simulink model "airship"  (Simulink 7.5)
settings: Solver=ode45  StartTime=0.0  StopTime=2  RelTol=1e-3
values from neighbouring files (symbols this model uses):
  a1 = 5    [valuables.m]
  a2 = 2*a1    (= 10)    [valuables.m]
  b = 3.7/2    (= 1.85)    [valuables.m]
  bottom = 0    [valuables.m]
  CL1 = (1/2)*DiffCLZeta*Sf*Nf*Lf3    (= 2.0002634928)    [valuables.m]
  CL2 = -Cdcg*Sg*Lgz    (= -1.344)    [valuables.m]
  CM1 = K21*Nk*Sh*I2*L    (= 217.968531349)    [valuables.m]
  CM2 = (-1/2)*DiffCLAlpha*Sf*Nf*Lf1    (= -59.34811401)    [valuables.m]
  CM3 = -((Cdch*J2*Sh*L)+(Cdcf*Sf*Lf2))    (= -168.6714915)    [valuables.m]
  CM4 = (-1/2)*DiffCLZeta*Sf*Nf*Lf1    (= -12.84322188)    [valuables.m]
  CX1 = -(Cdh0*Sh+Cdf0*Sf+Cdg0*Sg)    (= -0.6313245)    [valuables.m]
  CY1 = K21*Nk*Sh*I1    (= -6.9497212894)    [valuables.m]
  CY2 = (-1/2)*DiffCLAlpha*Sf*Nf    (= -8.4181722)    [valuables.m]
  CY3 = -((Cdch*J1*Sh)+(Cdcf*Sf)+(Cdcg*Sg))    (= -25.4932315)    [valuables.m]
  CY4 = (-1/2)*DiffCLZeta*Sf*Nf    (= -1.8217336)    [valuables.m]
  CZ3 = -((Cdch*J1*Sh)+(Cdcf*Sf))    (= -24.9332315)    [valuables.m]
  del = (Ixx*Izz)-(Ixz*Ixz)    (= 676199)    [valuables.m]
  g = 0.0669    [valuables.m]
  h0 = 200    [valuables.m]
  Ixx = 213    [valuables.m]
  Ixz = 88    [valuables.m]
  Iyy = 3310    [valuables.m]
  Izz = 3211    [valuables.m]
  left = 0    [valuables.m]
  mass = 136.8    [valuables.m]
  right = 0    [valuables.m]
  TL = 0.3    [valuables.m]
  top = 0    [valuables.m]
  TR = 0.3    [valuables.m]
  TS = 0.3    [valuables.m]
  u0 = 10    [valuables.m]
  XL = 8.13    [valuables.m]
  Xs = 12.5    [valuables.m]
  YL = 0.6    [valuables.m]
  ZL = 0.2    [valuables.m]
  Zs = 0.25    [valuables.m]
libraries: vrlib x2
settings Model: Creator=knightofaccess  LastModifiedBy=ex08148

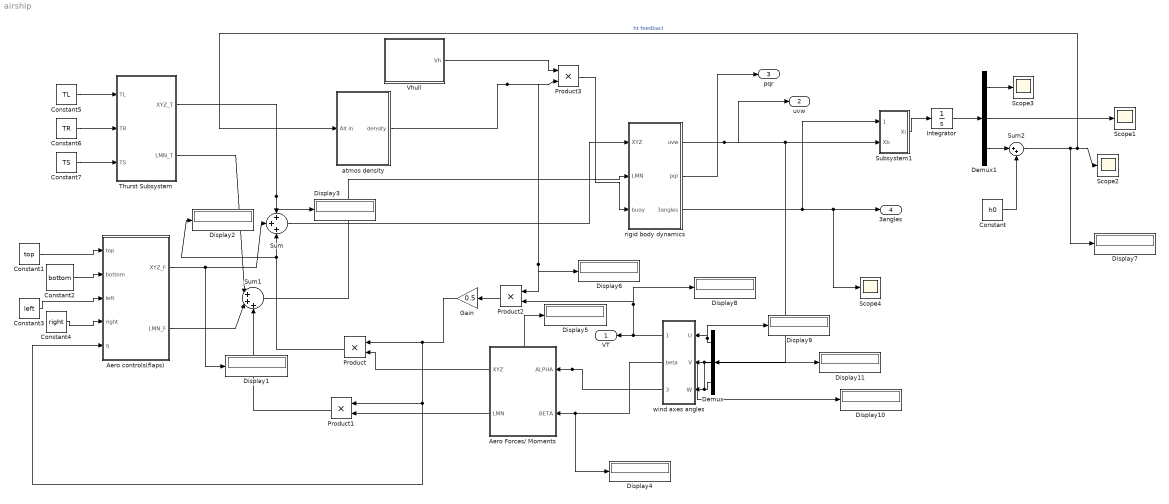
== system airship ==
  Aero Forces/ Moments : Subsystem
  Aero controls(flaps) : Subsystem
  Constant : Constant  Value=h0  OutDataType=fixdt(1, 16)  OutScaling=2^0
  Constant1 : Constant  Value=top  OutDataType=fixdt(1, 16)  OutScaling=2^0
  Constant2 : Constant  Value=bottom  OutDataType=fixdt(1, 16)  OutScaling=2^0
  Constant3 : Constant  Value=left  OutDataType=fixdt(1, 16)  OutScaling=2^0
  Constant4 : Constant  Value=right  OutDataType=fixdt(1, 16)  OutScaling=2^0
  Constant5 : Constant  Value=TL  OutDataType=fixdt(1, 16)  OutScaling=2^0
  Constant6 : Constant  Value=TR  OutDataType=fixdt(1, 16)  OutScaling=2^0
  Constant7 : Constant  Value=TS  OutDataType=fixdt(1, 16)  OutScaling=2^0
  Demux : Demux  Outputs=3
  Demux1 : Demux  Outputs=3
  Display{1..11} (11 alike) : Display
  Gain : Gain  Gain=0.5  ParameterDataType=fixdt(1, 16)  ParameterScaling=2^0  OutDataType=fixdt(1, 16)  OutScaling=2^0
  Integrator : Integrator
  Product{,1..3} (4 alike) : Product  OutDataType=fixdt(1, 16)  OutScaling=2^0  RndMeth=Zero
  Scope{1..4} (4 alike) : Scope
      Scope2 settings: SaveName=ScopeData2
      Scope4 settings: SaveName=ScopeData3
  Subsystem1 : Subsystem
  Sum : Sum  Inputs=+++  OutDataType=fixdt(1, 16)  OutScaling=2^0
  Sum1 : Sum  Inputs=|+++  OutDataType=fixdt(1, 16)  OutScaling=2^0
  Sum2 : Sum  Inputs=|++  OutDataType=fixdt(1, 16)  OutScaling=2^0
  Thurst Subsystem : Subsystem
  Vhull : Subsystem
  atmos density : Subsystem
  rigid body dynamics : Subsystem
  wind axes angles : Subsystem
  VT : Outport  OutDataType=fixdt(1, 16)  OutScaling=2^0
  uvw : Outport  Port=2
  pqr : Outport  Port=3
  3angles : Outport  Port=4
  wires:
  Thurst Subsystem/1(XYZ_T) -> Sum/1, Display3/1
  Thurst Subsystem/2(LMN_T) -> Sum1/1
  Constant5/1 -> Thurst Subsystem/1(TL)
  Constant6/1 -> Thurst Subsystem/2(TR)
  Constant7/1 -> Thurst Subsystem/3(TS)
  Aero controls(flaps)/2(LMN_F) -> Sum1/2
  Constant1/1 -> Aero controls(flaps)/1(top)
  Constant2/1 -> Aero controls(flaps)/2(bottom)
  Constant3/1 -> Aero controls(flaps)/3(left)
  Constant4/1 -> Aero controls(flaps)/4(right)
  Aero controls(flaps)/1(XYZ_F) -> Sum/2, Display1/1
  Aero Forces/ Moments/1(XYZ) -> Product/2
  Aero Forces/ Moments/2(LMN) -> Product1/2
  Product1/1 -> Sum1/3
  Product/1 -> Sum/3, Display2/1
  Demux/1 -> wind axes angles/1(U), Display9/1
  Demux/2 -> wind axes angles/2(V), Display10/1
  wind axes angles/1(VT*VT) -> VT/1, Product2/2, Display8/1
  wind axes angles/2(beta) -> Aero Forces/ Moments/2(BETA), Display4/1
  wind axes angles/3(alpha) -> Aero Forces/ Moments/1(ALPHA), Display5/1
  Product2/1 -> Gain/1
  Gain/1 -> Product/1, Aero controls(flaps)/5(q), Product1/1
  rigid body dynamics/1(uvw) -> uvw/1, Subsystem1/2(Xb), Demux/1
  rigid body dynamics/2(pqr) -> pqr/1
  Sum/1 -> rigid body dynamics/1(XYZ)
  Sum1/1 -> rigid body dynamics/2(LMN)
  rigid body dynamics/3(3angles) -> Subsystem1/1(3angles), 3angles/1, Scope4/1
  Vhull/1(Vh) -> Product3/1
  atmos density/1(density) -> Product3/2, Product2/1, Display6/1
  Product3/1 -> rigid body dynamics/3(buoy)
  Demux/3 -> wind axes angles/3(W), Display11/1
  Subsystem1/1(Xi) -> Integrator/1
  Integrator/1 -> Demux1/1
  Demux1/1 -> Scope3/1
  Demux1/2 -> Scope1/1
  Demux1/3 -> Sum2/1
  Constant/1 -> Sum2/2
  Sum2/1 -> atmos density/1(Alt in), Scope2/1, Display7/1  "ht feedbacl"

== system airship/Aero Forces/ Moments ==
  ALPHA : Inport  OutDataType=sfix(16)  OutScaling=2^0
  BETA : Inport  Port=2  OutDataType=sfix(16)  OutScaling=2^0
  Subsystem : Subsystem
  Subsystem1 : Subsystem
  XYZ : Outport  OutDataType=sfix(16)  OutScaling=2^0
  LMN : Outport  Port=2  OutDataType=sfix(16)  OutScaling=2^0
  wires:
  Subsystem/1(XYZ) -> XYZ/1
  Subsystem1/1(LMN) -> LMN/1
  ALPHA/1 -> Subsystem/1(ALPHA), Subsystem1/2(ALPHA)  "ALPHA"
  BETA/1 -> Subsystem/2(BETA), Subsystem1/1(BETA)  "BETA"

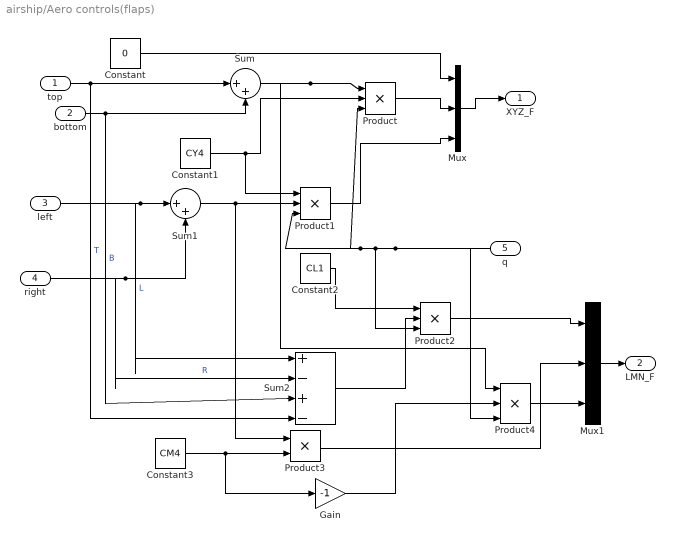
== system airship/Aero controls(flaps) ==
  top : Inport  OutDataType=sfix(16)  OutScaling=2^0
  bottom : Inport  Port=2  OutDataType=sfix(16)  OutScaling=2^0
  left : Inport  Port=3  OutDataType=sfix(16)  OutScaling=2^0
  right : Inport  Port=4  OutDataType=sfix(16)  OutScaling=2^0
  q : Inport  Port=5  OutDataType=fixdt(1, 16)  OutScaling=2^0
  Constant : Constant  Value=0  OutDataType=sfix(16)  OutScaling=2^0
  Constant1 : Constant  Value=CY4  OutDataType=sfix(16)  OutScaling=2^0
  Constant2 : Constant  Value=CL1  OutDataType=sfix(16)  OutScaling=2^0
  Constant3 : Constant  Value=CM4  OutDataType=sfix(16)  OutScaling=2^0
  Gain : Gain  Gain=-1  ParameterDataType=sfix(16)  ParameterScaling=2^0  OutDataType=sfix(16)  OutScaling=2^0
  Mux : Mux  Inputs=3
  Mux1 : Mux  Inputs=3
  Product{,1..2,4} (4 alike) : Product  Inputs=3  OutDataType=sfix(16)  OutScaling=2^0  RndMeth=Zero
  Product3 : Product  OutDataType=sfix(16)  OutScaling=2^0  RndMeth=Zero
  Sum : Sum  Inputs=|++  OutDataType=sfix(16)  OutScaling=2^0
  Sum1 : Sum  Inputs=|++  OutDataType=sfix(16)  OutScaling=2^0
  Sum2 : Sum  Inputs=|+-+-  OutDataType=sfix(16)  OutScaling=2^0
  XYZ_F : Outport  OutDataType=sfix(16)  OutScaling=2^0
  LMN_F : Outport  Port=2  OutDataType=sfix(16)  OutScaling=2^0
  wires:
  top/1 -> Sum/1, Sum2/4  "T"
  bottom/1 -> Sum/2, Sum2/3  "B"
  Sum/1 -> Product/1, Product4/1
  Constant1/1 -> Product/2, Product1/1
  left/1 -> Sum1/1, Sum2/1  "L"
  right/1 -> Sum1/2, Sum2/2  "R"
  Sum1/1 -> Product1/2, Product3/1
  Constant/1 -> Mux/1
  Product/1 -> Mux/2
  Product1/1 -> Mux/3
  Sum2/1 -> Product2/2
  Constant2/1 -> Product2/1
  Constant3/1 -> Product3/2, Gain/1
  Product4/1 -> Mux1/3
  Product3/1 -> Mux1/2
  Product2/1 -> Mux1/1
  Mux1/1 -> LMN_F/1
  Gain/1 -> Product4/2
  q/1 -> Product1/3, Product/3, Product4/3, Product2/3
  Mux/1 -> XYZ_F/1

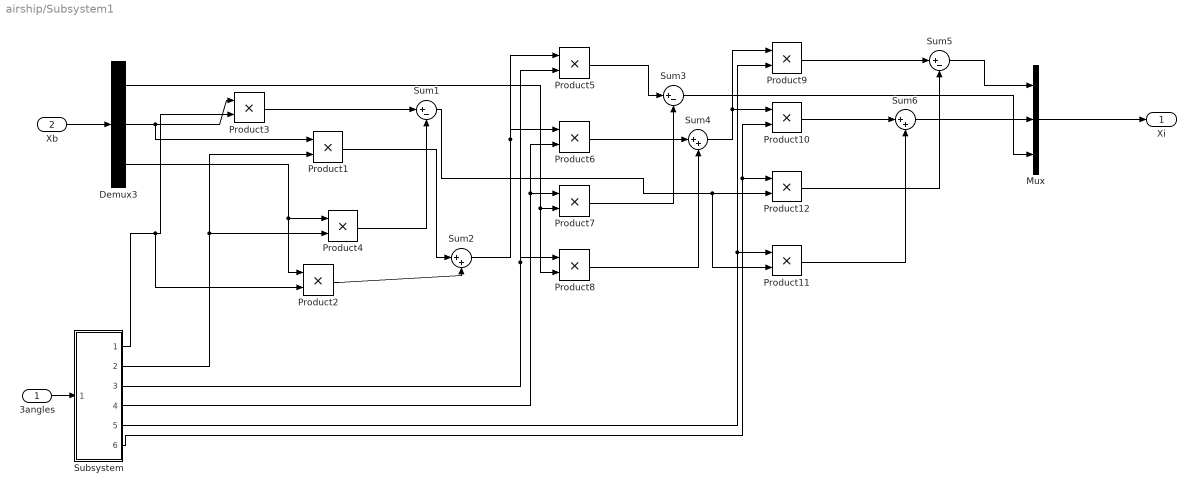
== system airship/Subsystem1 ==
  3angles : Inport  OutDataType=sfix(16)  OutScaling=2^0
  Xb : Inport  Port=2  OutDataType=sfix(16)  OutScaling=2^0
  Demux3 : Demux  Outputs=3
  Mux : Mux  Inputs=3
  Product{1..12} (12 alike) : Product  OutDataType=fixdt(1, 16)  OutScaling=2^0  RndMeth=Zero
  Subsystem : Subsystem
  Sum1 : Sum  Inputs=|+-  OutDataType=fixdt(1, 16)  OutScaling=2^0
  Sum2 : Sum  Inputs=|++  OutDataType=fixdt(1, 16)  OutScaling=2^0
  Sum3 : Sum  Inputs=|+-  OutDataType=fixdt(1, 16)  OutScaling=2^0
  Sum4 : Sum  Inputs=|++  OutDataType=fixdt(1, 16)  OutScaling=2^0
  Sum5 : Sum  Inputs=|+-  OutDataType=fixdt(1, 16)  OutScaling=2^0
  Sum6 : Sum  Inputs=|++  OutDataType=fixdt(1, 16)  OutScaling=2^0
  Xi : Outport  OutDataType=fixdt(1, 16)  OutScaling=2^0
  wires:
  3angles/1 -> Subsystem/1(3angles)
  Xb/1 -> Demux3/1
  Demux3/2 -> Product3/1, Product1/1
  Subsystem/1(cphi) -> Product3/2, Product2/2
  Subsystem/2(sphi) -> Product1/2, Product4/2
  Demux3/3 -> Product2/1, Product4/1
  Product4/1 -> Sum1/2
  Product2/1 -> Sum2/2
  Product3/1 -> Sum1/1
  Product1/1 -> Sum2/1
  Sum2/1 -> Product5/1, Product6/1
  Subsystem/3(ctheta) -> Product5/2, Product8/1
  Subsystem/4(stheta) -> Product6/2, Product7/1
  Demux3/1 -> Product7/2, Product8/2
  Product5/1 -> Sum3/1
  Product7/1 -> Sum3/2
  Product6/1 -> Sum4/1
  Product8/1 -> Sum4/2
  Sum4/1 -> Product9/1, Product10/1
  Subsystem/5(cpsi) -> Product9/2, Product11/1
  Subsystem/6(spsi) -> Product10/2, Product12/1
  Sum1/1 -> Product12/2, Product11/2
  Product9/1 -> Sum5/1
  Product12/1 -> Sum5/2
  Product10/1 -> Sum6/1
  Product11/1 -> Sum6/2
  Sum5/1 -> Mux/1
  Sum6/1 -> Mux/2
  Sum3/1 -> Mux/3
  Mux/1 -> Xi/1

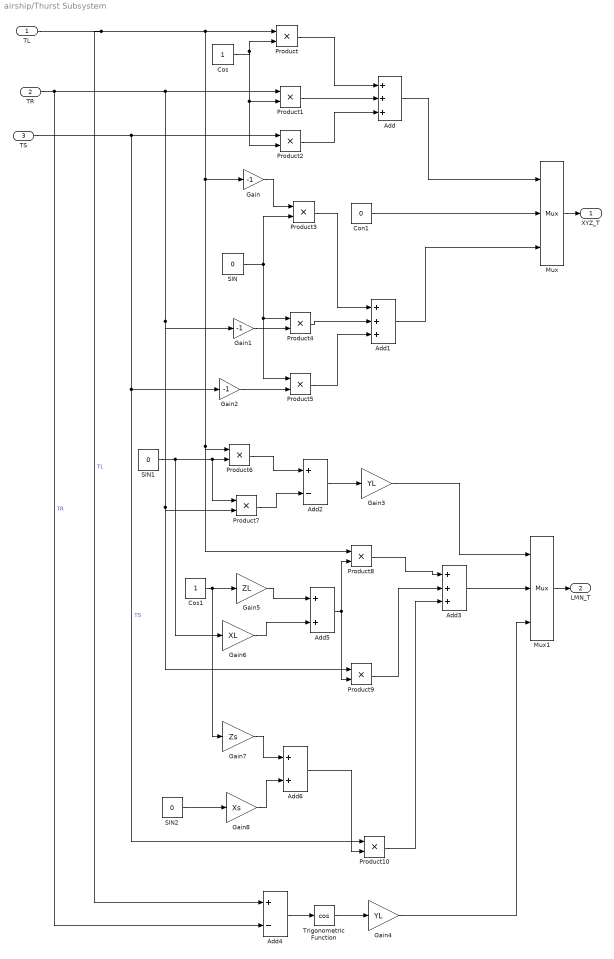
== system airship/Thurst Subsystem ==
  TL : Inport  OutDataType=sfix(16)  OutScaling=2^0
  TR : Inport  Port=2  OutDataType=sfix(16)  OutScaling=2^0
  TS : Inport  Port=3  OutDataType=sfix(16)  OutScaling=2^0
  Add : Sum  Inputs=+++  OutDataType=sfix(16)  OutScaling=2^-10
  Add1 : Sum  Inputs=+++  OutDataType=sfix(16)  OutScaling=2^-10
  Add2 : Sum  Inputs=+-  OutDataType=sfix(16)  OutScaling=2^-10
  Add3 : Sum  Inputs=+++  OutDataType=sfix(16)  OutScaling=2^-10
  Add4 : Sum  Inputs=+-  OutDataType=sfix(16)  OutScaling=2^-10
  Add5 : Sum  OutDataType=sfix(16)  OutScaling=2^-10
  Add6 : Sum  OutDataType=sfix(16)  OutScaling=2^-10
  Con1 : Constant  Value=0  OutDataType=sfix(16)  OutScaling=2^0
  Cos : Constant  OutDataType=sfix(16)  OutScaling=2^0
  Cos1 : Constant  OutDataType=sfix(16)  OutScaling=2^0
  Gain : Gain  Gain=-1  ParameterDataType=sfix(16)  ParameterScaling=2^0  OutDataType=sfix(16)  OutScaling=2^0
  Gain1 : Gain  Gain=-1  ParameterDataType=sfix(16)  ParameterScaling=2^0  OutDataType=sfix(16)  OutScaling=2^0
  Gain2 : Gain  Gain=-1  ParameterDataType=sfix(16)  ParameterScaling=2^0  OutDataType=sfix(16)  OutScaling=2^0
  Gain3 : Gain  Gain=YL  ParameterDataType=sfix(16)  ParameterScaling=2^0  OutDataType=sfix(16)  OutScaling=2^0
  Gain4 : Gain  Gain=YL  ParameterDataType=sfix(16)  ParameterScaling=2^0  OutDataType=sfix(16)  OutScaling=2^0
  Gain5 : Gain  Gain=ZL  ParameterDataType=sfix(16)  ParameterScaling=2^0  OutDataType=sfix(16)  OutScaling=2^0
  Gain6 : Gain  Gain=XL  ParameterDataType=sfix(16)  ParameterScaling=2^0  OutDataType=sfix(16)  OutScaling=2^0
  Gain7 : Gain  Gain=Zs  ParameterDataType=sfix(16)  ParameterScaling=2^0  OutDataType=sfix(16)  OutScaling=2^0
  Gain8 : Gain  Gain=Xs  ParameterDataType=sfix(16)  ParameterScaling=2^0  OutDataType=sfix(16)  OutScaling=2^0
  Mux : Mux  Inputs=3
  Mux1 : Mux  Inputs=3
  Product{,1..10} (11 alike) : Product  OutDataType=sfix(16)  OutScaling=2^0  RndMeth=Zero
  SIN : Constant  Value=0  OutDataType=sfix(16)  OutScaling=2^0
  SIN1 : Constant  Value=0  OutDataType=sfix(16)  OutScaling=2^0
  SIN2 : Constant  Value=0  OutDataType=sfix(16)  OutScaling=2^0
  Trigonometric Function : Trigonometry  Operator=cos  SampleTime=0
  XYZ_T : Outport  OutDataType=sfix(16)  OutScaling=2^0
  LMN_T : Outport  Port=2  OutDataType=sfix(16)  OutScaling=2^0
  wires:
  TL/1 -> Product/1, Gain/1, Product6/1, Product8/1, Add4/1  "TL"
  Cos/1 -> Product/2, Product1/2, Product2/2
  TR/1 -> Product1/1, Gain1/1, Product7/2, Product9/1, Add4/2  "TR"
  TS/1 -> Product2/1, Gain2/1, Product10/1  "TS"
  Product/1 -> Add/1
  Product1/1 -> Add/2
  Product2/1 -> Add/3
  SIN/1 -> Product3/2, Product4/1, Product5/1
  Gain/1 -> Product3/1
  Gain1/1 -> Product4/2
  Gain2/1 -> Product5/2
  Product3/1 -> Add1/1
  Product4/1 -> Add1/2
  Product5/1 -> Add1/3
  Add/1 -> Mux/1
  Con1/1 -> Mux/2
  Add1/1 -> Mux/3
  SIN1/1 -> Product6/2, Product7/1, Gain6/1
  Product6/1 -> Add2/1
  Product7/1 -> Add2/2
  Add2/1 -> Gain3/1
  Gain3/1 -> Mux1/1
  Product8/1 -> Add3/1
  Product9/1 -> Add3/2
  Product10/1 -> Add3/3
  Add3/1 -> Mux1/2
  Gain4/1 -> Mux1/3
  Mux/1 -> XYZ_T/1
  Mux1/1 -> LMN_T/1
  Gain5/1 -> Add5/1
  Cos1/1 -> Gain5/1, Gain7/1
  Gain6/1 -> Add5/2
  Add5/1 -> Product8/2, Product9/2
  SIN2/1 -> Gain8/1
  Gain7/1 -> Add6/1
  Gain8/1 -> Add6/2
  Add6/1 -> Product10/2
  Trigonometric Function/1 -> Gain4/1
  Add4/1 -> Trigonometric Function/1

== system airship/Vhull ==
  Constant : Constant  Value=a1  OutDataType=sfix(16)  OutScaling=2^0
  Constant1 : Constant  Value=a2  OutDataType=sfix(16)  OutScaling=2^0
  Constant2 : Constant  Value=b*b  OutDataType=sfix(16)  OutScaling=2^0
  Gain : Gain  Gain=pi*2/3  ParameterDataType=sfix(16)  ParameterScaling=2^0  OutDataType=sfix(16)  OutScaling=2^0
  Product : Product  OutDataType=sfix(16)  OutScaling=2^0  RndMeth=Zero
  Subtract : Sum  OutDataType=sfix(16)  OutScaling=2^-10
  Vh : Outport  OutDataType=sfix(16)  OutScaling=2^0
  wires:
  Constant/1 -> Subtract/1
  Constant1/1 -> Subtract/2
  Subtract/1 -> Product/1
  Constant2/1 -> Product/2
  Product/1 -> Gain/1
  Gain/1 -> Vh/1

== system airship/atmos density ==
  Alt in : Inport  OutDataType=sfix(16)  OutScaling=2^0
  Constant : Constant  Value=0.0065  OutDataType=sfix(16)  OutScaling=2^0
  Constant1 : Constant  Value=288.15  OutDataType=sfix(16)  OutScaling=2^0
  Display1 : Display
  Divide1 : Product  Inputs=*/  OutDataType=fixdt(1, 16)  OutScaling=2^-10
  Fcn : Fcn  Expr=u^4.256
  Gain : Gain  Gain=1.22505  ParameterDataType=sfix(16)  ParameterScaling=2^0  OutDataType=sfix(16)  OutScaling=2^0
  Product : Product  OutDataType=sfix(16)  OutScaling=2^0  RndMeth=Zero
  Sum2 : Sum  Inputs=|-+
  density : Outport  OutDataType=sfix(16)  OutScaling=2^0
  wires:
  Constant/1 -> Product/2
  Product/1 -> Sum2/1
  Constant1/1 -> Sum2/2, Divide1/2
  Divide1/1 -> Fcn/1
  Fcn/1 -> Gain/1, Display1/1
  Alt in/1 -> Product/1
  Gain/1 -> density/1
  Sum2/1 -> Divide1/1

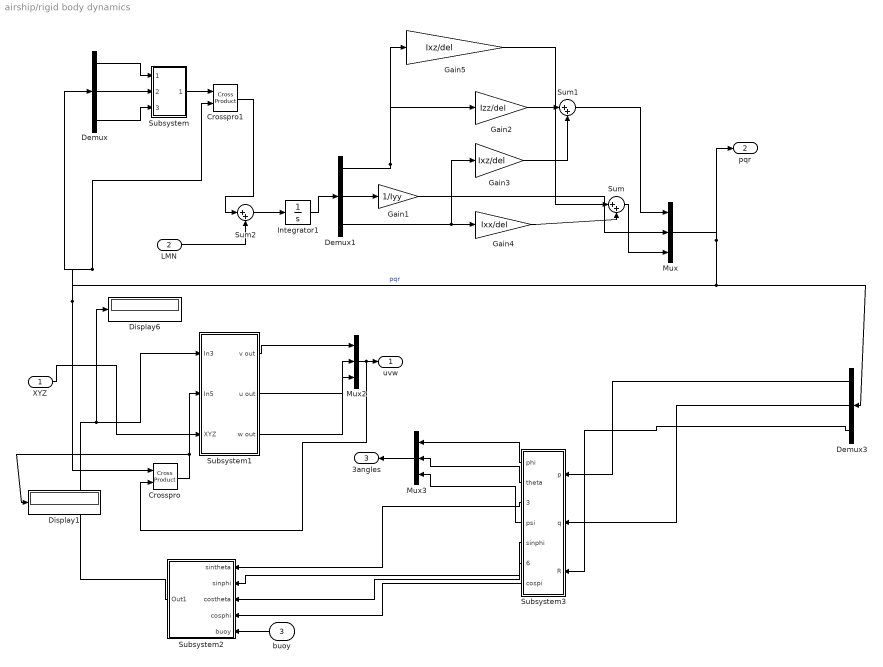
== system airship/rigid body dynamics ==
  XYZ : Inport
  LMN : Inport  Port=2
  buoy : Inport  Port=3
  Crosspro : vrlib/Utilities/Cross Product  SystemSampleTime=-1
  Crosspro1 : vrlib/Utilities/Cross Product  SystemSampleTime=-1
  Demux : Demux  Outputs=3
  Demux1 : Demux  Outputs=3
  Demux3 : Demux  Outputs=3
  Display1 : Display
  Display6 : Display
  Gain1 : Gain  Gain=1/Iyy
  Gain2 : Gain  Gain=Izz/del
  Gain3 : Gain  Gain=Ixz/del
  Gain4 : Gain  Gain=Ixx/del
  Gain5 : Gain  Gain=Ixz/del
  Integrator1 : Integrator
  Mux : Mux  Inputs=3
  Mux2 : Mux  Inputs=3
  Mux3 : Mux  Inputs=3
  Subsystem : Subsystem
  Subsystem1 : Subsystem
  Subsystem2 : Subsystem
  Subsystem3 : Subsystem
  Sum : Sum  Inputs=|++
  Sum1 : Sum  Inputs=|++
  Sum2 : Sum  Inputs=|++
  uvw : Outport
  pqr : Outport  Port=2
  3angles : Outport  Port=3
  wires:
  Mux3/1 -> 3angles/1
  Mux2/1 -> uvw/1, Crosspro/2
  Demux/2 -> Subsystem/2(In2)
  Demux/1 -> Subsystem/1(In1)
  Demux/3 -> Subsystem/3(In3)
  Demux1/1 -> Gain5/1, Gain2/1
  Demux1/2 -> Gain1/1
  Demux1/3 -> Gain4/1, Gain3/1
  Gain4/1 -> Sum/2
  Gain5/1 -> Sum/1
  Gain2/1 -> Sum1/1
  Gain3/1 -> Sum1/2
  Gain1/1 -> Mux/2
  Sum1/1 -> Mux/1
  Sum/1 -> Mux/3
  Mux/1 -> Demux/1, Crosspro1/2, Crosspro/1, Demux3/1, pqr/1  "pqr"
  Subsystem/1(Out1) -> Crosspro1/1
  Crosspro1/1 -> Sum2/1
  Sum2/1 -> Integrator1/1
  Integrator1/1 -> Demux1/1
  Crosspro/1 -> Subsystem1/2(In5), Display1/1
  Subsystem1/1(v out) -> Mux2/1
  Subsystem1/2(u out) -> Mux2/2
  Subsystem1/3(w out) -> Mux2/3
  Subsystem2/1(Out1) -> Subsystem1/1(In3), Display6/1
  Subsystem3/1(phi) -> Mux3/1
  Subsystem3/2(theta) -> Mux3/2
  Demux3/1 -> Subsystem3/1(p)
  Demux3/2 -> Subsystem3/2(q)
  Demux3/3 -> Subsystem3/3(R)
  Subsystem3/3(sinthta) -> Subsystem2/1(sintheta)
  Subsystem3/4(psi) -> Mux3/3
  Subsystem3/6(costhta) -> Subsystem2/3(costheta)
  Subsystem3/7(cospi) -> Subsystem2/4(cosphi)
  Subsystem3/5(sinphi) -> Subsystem2/2(sinphi)
  XYZ/1 -> Subsystem1/3(XYZ)
  LMN/1 -> Sum2/2
  buoy/1 -> Subsystem2/5(buoy)

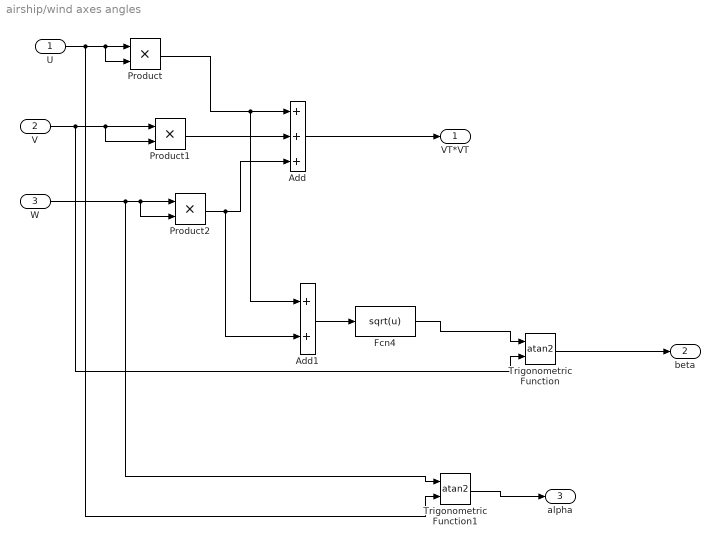
== system airship/wind axes angles ==
  U : Inport  OutDataType=fixdt(1, 16)  OutScaling=2^0
  V : Inport  Port=2  OutDataType=fixdt(1, 16)  OutScaling=2^0
  W : Inport  Port=3  OutDataType=fixdt(1, 16)  OutScaling=2^0
  Add : Sum  Inputs=+++  OutDataType=fixdt(1, 16)  OutScaling=2^-10
  Add1 : Sum  OutDataType=fixdt(1, 16)  OutScaling=2^-10
  Fcn4 : Fcn  Expr=sqrt(u)
  Product : Product  OutDataType=fixdt(1, 16)  OutScaling=2^0  RndMeth=Zero
  Product1 : Product  OutDataType=fixdt(1, 16)  OutScaling=2^0  RndMeth=Zero
  Product2 : Product  OutDataType=fixdt(1, 16)  OutScaling=2^0  RndMeth=Zero
  Trigonometric Function : Trigonometry  Operator=atan2
  Trigonometric Function1 : Trigonometry  Operator=atan2
  VT*VT : Outport  OutDataType=fixdt(1, 16)  OutScaling=2^0
  beta : Outport  Port=2  OutDataType=fixdt(1, 16)  OutScaling=2^0
  alpha : Outport  Port=3  OutDataType=fixdt(1, 16)  OutScaling=2^0
  wires:
  U/1 -> Product/1, Product/2, Trigonometric Function1/2
  V/1 -> Product1/1, Product1/2, Trigonometric Function/2
  W/1 -> Product2/1, Product2/2, Trigonometric Function1/1
  Product/1 -> Add/1, Add1/1
  Product1/1 -> Add/2
  Product2/1 -> Add/3, Add1/2
  Add1/1 -> Fcn4/1
  Fcn4/1 -> Trigonometric Function/1
  Add/1 -> VT*VT/1
  Trigonometric Function1/1 -> alpha/1
  Trigonometric Function/1 -> beta/1

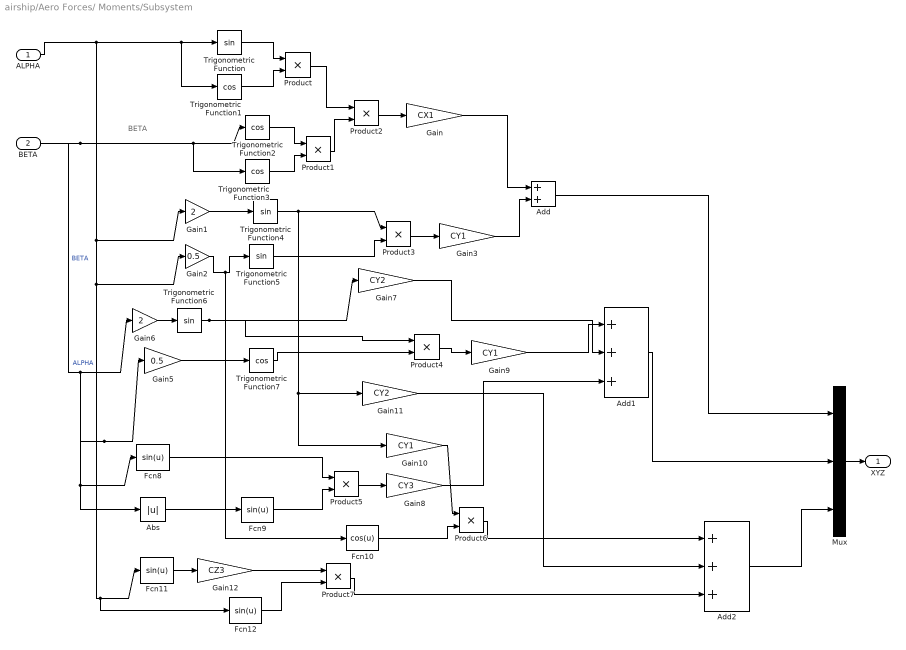
== system airship/Aero Forces/ Moments/Subsystem ==
  note: BETA
  ALPHA : Inport  OutDataType=sfix(16)  OutScaling=2^0
  BETA : Inport  Port=2  OutDataType=sfix(16)  OutScaling=2^0
  Abs : Abs
  Add : Sum  OutDataType=sfix(16)  OutScaling=2^-10
  Add1 : Sum  Inputs=+++  OutDataType=sfix(16)  OutScaling=2^-10
  Add2 : Sum  Inputs=+++  OutDataType=sfix(16)  OutScaling=2^-10
  Fcn10 : Fcn  Expr=cos(u)
  Fcn{8..9,11..12} (4 alike) : Fcn  Expr=sin(u)
  Gain : Gain  Gain=CX1  ParameterDataType=sfix(16)  ParameterScaling=2^0  OutDataType=sfix(16)  OutScaling=2^0
  Gain1 : Gain  Gain=2  ParameterDataType=sfix(16)  ParameterScaling=2^0  OutDataType=sfix(16)  OutScaling=2^0
  Gain10 : Gain  Gain=CY1  ParameterDataType=sfix(16)  ParameterScaling=2^0  OutDataType=sfix(16)  OutScaling=2^0
  Gain11 : Gain  Gain=CY2  ParameterDataType=sfix(16)  ParameterScaling=2^0  OutDataType=sfix(16)  OutScaling=2^0
  Gain12 : Gain  Gain=CZ3  ParameterDataType=sfix(16)  ParameterScaling=2^0  OutDataType=sfix(16)  OutScaling=2^0
  Gain2 : Gain  Gain=0.5  ParameterDataType=sfix(16)  ParameterScaling=2^0  OutDataType=sfix(16)  OutScaling=2^0
  Gain3 : Gain  Gain=CY1  ParameterDataType=sfix(16)  ParameterScaling=2^0  OutDataType=sfix(16)  OutScaling=2^0
  Gain5 : Gain  Gain=0.5  ParameterDataType=sfix(16)  ParameterScaling=2^0  OutDataType=sfix(16)  OutScaling=2^0
  Gain6 : Gain  Gain=2  ParameterDataType=sfix(16)  ParameterScaling=2^0  OutDataType=sfix(16)  OutScaling=2^0
  Gain7 : Gain  Gain=CY2  ParameterDataType=sfix(16)  ParameterScaling=2^0  OutDataType=sfix(16)  OutScaling=2^0
  Gain8 : Gain  Gain=CY3  ParameterDataType=sfix(16)  ParameterScaling=2^0  OutDataType=sfix(16)  OutScaling=2^0
  Gain9 : Gain  Gain=CY1  ParameterDataType=sfix(16)  ParameterScaling=2^0  OutDataType=sfix(16)  OutScaling=2^0
  Mux : Mux  Inputs=3
  Product{,1..7} (8 alike) : Product  OutDataType=sfix(16)  OutScaling=2^0  RndMeth=Zero
  Trigonometric Function{,4..6} (4 alike) : Trigonometry
  Trigonometric Function{1..3,7} (4 alike) : Trigonometry  Operator=cos
  XYZ : Outport
  wires:
  ALPHA/1 -> Fcn11/1, Fcn12/1, Gain2/1, Gain1/1, Trigonometric Function/1, Trigonometric Function1/1  "ALPHA"
  BETA/1 -> Gain5/1, Abs/1, Fcn8/1, Gain6/1, Trigonometric Function2/1, Trigonometric Function3/1  "BETA"
  Add2/1 -> Mux/3
  Add1/1 -> Mux/2
  Add/1 -> Mux/1
  Product7/1 -> Add2/3
  Gain11/1 -> Add2/2
  Product6/1 -> Add2/1
  Fcn12/1 -> Product7/2
  Fcn10/1 -> Product6/2
  Gain10/1 -> Product6/1
  Gain8/1 -> Add1/3
  Gain7/1 -> Add1/2
  Product5/1 -> Gain8/1
  Fcn9/1 -> Product5/2
  Fcn8/1 -> Product5/1
  Abs/1 -> Fcn9/1
  Trigonometric Function7/1 -> Product4/2
  Gain6/1 -> Trigonometric Function6/1
  Trigonometric Function6/1 -> Gain7/1, Product4/1
  Gain5/1 -> Trigonometric Function7/1
  Gain3/1 -> Add/2
  Gain/1 -> Add/1
  Product3/1 -> Gain3/1
  Trigonometric Function5/1 -> Product3/2
  Trigonometric Function4/1 -> Gain11/1, Gain10/1, Product3/1
  Gain2/1 -> Fcn10/1, Trigonometric Function5/1
  Gain1/1 -> Trigonometric Function4/1
  Product2/1 -> Gain/1
  Product1/1 -> Product2/2
  Product/1 -> Product2/1
  Trigonometric Function3/1 -> Product1/2
  Trigonometric Function2/1 -> Product1/1
  Trigonometric Function1/1 -> Product/2
  Trigonometric Function/1 -> Product/1
  Fcn11/1 -> Gain12/1
  Gain12/1 -> Product7/1
  Mux/1 -> XYZ/1
  Gain9/1 -> Add1/1
  Product4/1 -> Gain9/1

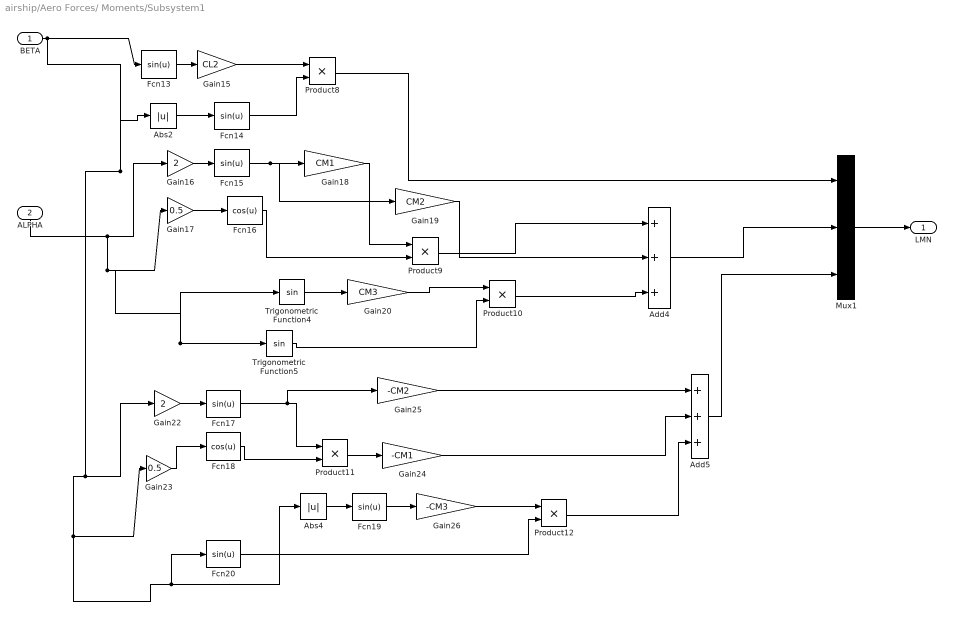
== system airship/Aero Forces/ Moments/Subsystem1 ==
  BETA : Inport
  ALPHA : Inport  Port=2
  Abs2 : Abs
  Abs4 : Abs
  Add4 : Sum  Inputs=+++  OutDataType=sfix(16)  OutScaling=2^-10
  Add5 : Sum  Inputs=+++  OutDataType=sfix(16)  OutScaling=2^-10
  Fcn{13..15,17,19..20} (6 alike) : Fcn  Expr=sin(u)
  Fcn16 : Fcn  Expr=cos(u)
  Fcn18 : Fcn  Expr=cos(u)
  Gain15 : Gain  Gain=CL2  ParameterDataType=sfix(16)  ParameterScaling=2^0  OutDataType=sfix(16)  OutScaling=2^0
  Gain16 : Gain  Gain=2  ParameterDataType=sfix(16)  ParameterScaling=2^0  OutDataType=sfix(16)  OutScaling=2^0
  Gain17 : Gain  Gain=0.5  ParameterDataType=sfix(16)  ParameterScaling=2^0  OutDataType=sfix(16)  OutScaling=2^0
  Gain18 : Gain  Gain=CM1  ParameterDataType=sfix(16)  ParameterScaling=2^0  OutDataType=sfix(16)  OutScaling=2^0
  Gain19 : Gain  Gain=CM2  ParameterDataType=sfix(16)  ParameterScaling=2^0  OutDataType=sfix(16)  OutScaling=2^0
  Gain20 : Gain  Gain=CM3  ParameterDataType=sfix(16)  ParameterScaling=2^0  OutDataType=sfix(16)  OutScaling=2^0
  Gain22 : Gain  Gain=2  ParameterDataType=sfix(16)  ParameterScaling=2^0  OutDataType=sfix(16)  OutScaling=2^0
  Gain23 : Gain  Gain=0.5  ParameterDataType=sfix(16)  ParameterScaling=2^0  OutDataType=sfix(16)  OutScaling=2^0
  Gain24 : Gain  Gain=-CM1  ParameterDataType=sfix(16)  ParameterScaling=2^0  OutDataType=sfix(16)  OutScaling=2^0
  Gain25 : Gain  Gain=-CM2  ParameterDataType=sfix(16)  ParameterScaling=2^0  OutDataType=sfix(16)  OutScaling=2^0
  Gain26 : Gain  Gain=-CM3  ParameterDataType=sfix(16)  ParameterScaling=2^0  OutDataType=sfix(16)  OutScaling=2^0
  Mux1 : Mux  Inputs=3
  Product{8..12} (5 alike) : Product  OutDataType=sfix(16)  OutScaling=2^0  RndMeth=Zero
  Trigonometric Function4 : Trigonometry
  Trigonometric Function5 : Trigonometry
  LMN : Outport
  wires:
  Fcn13/1 -> Gain15/1
  Abs2/1 -> Fcn14/1
  Gain15/1 -> Product8/1
  Fcn14/1 -> Product8/2
  Product8/1 -> Mux1/1
  Gain16/1 -> Fcn15/1
  Gain17/1 -> Fcn16/1
  Fcn15/1 -> Gain19/1, Gain18/1
  Fcn16/1 -> Product9/2
  Gain18/1 -> Product9/1
  Trigonometric Function5/1 -> Product10/2
  Trigonometric Function4/1 -> Gain20/1
  Gain20/1 -> Product10/1
  Product9/1 -> Add4/1
  Gain19/1 -> Add4/2
  Product10/1 -> Add4/3
  Gain22/1 -> Fcn17/1
  Fcn17/1 -> Gain25/1, Product11/1
  Gain23/1 -> Fcn18/1
  Fcn18/1 -> Product11/2
  Product11/1 -> Gain24/1
  Abs4/1 -> Fcn19/1
  Fcn19/1 -> Gain26/1
  Fcn20/1 -> Product12/2
  Gain26/1 -> Product12/1
  Gain25/1 -> Add5/1
  Gain24/1 -> Add5/2
  Product12/1 -> Add5/3
  Add4/1 -> Mux1/2
  Add5/1 -> Mux1/3
  BETA/1 -> Fcn13/1, Gain23/1, Fcn20/1, Abs4/1, Gain22/1, Abs2/1
  ALPHA/1 -> Trigonometric Function4/1, Trigonometric Function5/1, Gain17/1, Gain16/1
  Mux1/1 -> LMN/1

== system airship/Subsystem1/Subsystem ==
  note: psi
  note: theta
  note: phi
  3angles : Inport  OutDataType=sfix(16)  OutScaling=2^0
  Demux2 : Demux  Outputs=3
  Trigonometric Function : Trigonometry
  Trigonometric Function1 : Trigonometry  Operator=cos
  Trigonometric Function2 : Trigonometry  Operator=cos
  Trigonometric Function3 : Trigonometry
  Trigonometric Function4 : Trigonometry  Operator=cos
  Trigonometric Function5 : Trigonometry
  cphi : Outport
  sphi : Outport  Port=2
  ctheta : Outport  Port=3
  stheta : Outport  Port=4
  cpsi : Outport  Port=5
  spsi : Outport  Port=6
  wires:
  Demux2/1 -> Trigonometric Function1/1, Trigonometric Function/1
  Demux2/2 -> Trigonometric Function2/1, Trigonometric Function3/1
  3angles/1 -> Demux2/1
  Demux2/3 -> Trigonometric Function4/1, Trigonometric Function5/1
  Trigonometric Function1/1 -> cphi/1
  Trigonometric Function/1 -> sphi/1
  Trigonometric Function2/1 -> ctheta/1
  Trigonometric Function3/1 -> stheta/1
  Trigonometric Function4/1 -> cpsi/1
  Trigonometric Function5/1 -> spsi/1

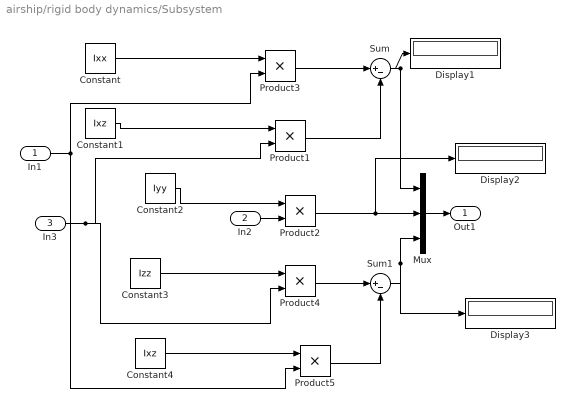
== system airship/rigid body dynamics/Subsystem ==
  In1 : Inport
  In2 : Inport  Port=2
  In3 : Inport  Port=3
  Constant : Constant  Value=Ixx
  Constant1 : Constant  Value=Ixz
  Constant2 : Constant  Value=Iyy
  Constant3 : Constant  Value=Izz
  Constant4 : Constant  Value=Ixz
  Display1 : Display
  Display2 : Display
  Display3 : Display
  Mux : Mux  Inputs=3
  Product{1..5} (5 alike) : Product  RndMeth=Zero
  Sum : Sum  Inputs=|+-
  Sum1 : Sum  Inputs=|+-
  Out1 : Outport
  wires:
  In1/1 -> Product5/2, Product3/2
  Constant4/1 -> Product5/1
  In3/1 -> Product1/2, Product4/2
  Constant3/1 -> Product4/1
  Constant2/1 -> Product2/1
  Constant1/1 -> Product1/1
  Constant/1 -> Product3/1
  Product3/1 -> Sum/1
  Product1/1 -> Sum/2
  Product4/1 -> Sum1/1
  Product5/1 -> Sum1/2
  Product2/1 -> Mux/2, Display2/1
  Sum1/1 -> Mux/3, Display3/1
  Sum/1 -> Mux/1, Display1/1
  Mux/1 -> Out1/1
  In2/1 -> Product2/2

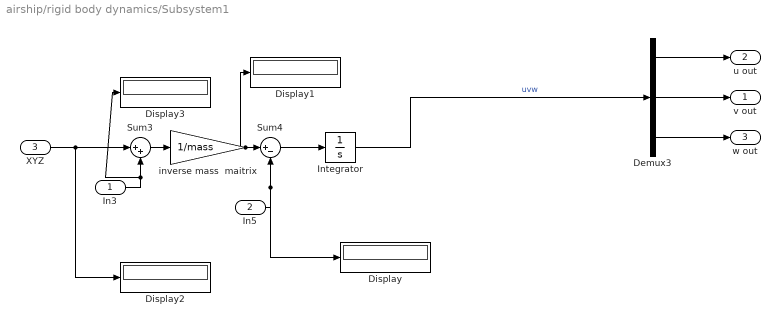
== system airship/rigid body dynamics/Subsystem1 ==
  In3 : Inport
  In5 : Inport  Port=2
  XYZ : Inport  Port=3
  Demux3 : Demux  Outputs=3
  Display{,1..3} (4 alike) : Display
  Integrator : Integrator  InitialCondition=[u0 0 0]'
  Sum3 : Sum  Inputs=|++
  Sum4 : Sum  Inputs=|+-
  inverse mass  maitrix : Gain  Gain=1/mass
  v out : Outport
  u out : Outport  Port=2
  w out : Outport  Port=3
  wires:
  Demux3/1 -> u out/1
  Demux3/2 -> v out/1
  Demux3/3 -> w out/1
  Integrator/1 -> Demux3/1  "uvw"
  Sum4/1 -> Integrator/1
  inverse mass  maitrix/1 -> Sum4/1, Display1/1
  Sum3/1 -> inverse mass  maitrix/1
  In3/1 -> Sum3/2, Display3/1
  In5/1 -> Sum4/2, Display/1
  XYZ/1 -> Sum3/1, Display2/1

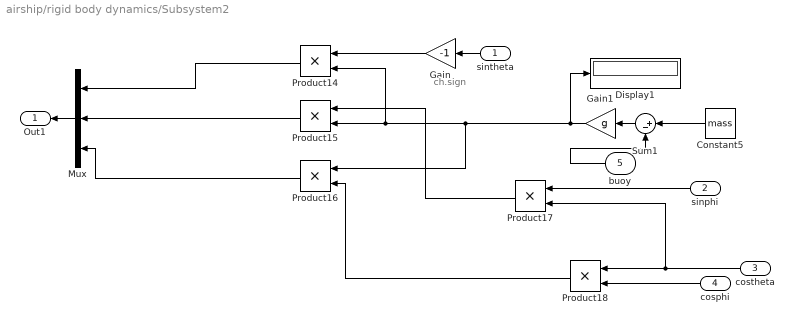
== system airship/rigid body dynamics/Subsystem2 ==
  note: ch.sign
  sintheta : Inport
  sinphi : Inport  Port=2
  costheta : Inport  Port=3
  cosphi : Inport  Port=4
  buoy : Inport  Port=5
  Constant5 : Constant  Value=mass
  Display1 : Display
  Gain : Gain  Gain=-1
  Gain1 : Gain  Gain=g
  Mux : Mux  Inputs=3
  Product{14..18} (5 alike) : Product  RndMeth=Zero
  Sum1 : Sum  Inputs=|+-
  Out1 : Outport
  wires:
  Product14/1 -> Mux/1
  Product15/1 -> Mux/2
  Product16/1 -> Mux/3
  Gain/1 -> Product14/1
  Product17/1 -> Product15/1
  Product18/1 -> Product16/2
  sinphi/1 -> Product17/1
  costheta/1 -> Product18/1, Product17/2
  cosphi/1 -> Product18/2
  sintheta/1 -> Gain/1
  Mux/1 -> Out1/1
  buoy/1 -> Sum1/2
  Gain1/1 -> Product16/1, Product15/2, Product14/2, Display1/1
  Sum1/1 -> Gain1/1
  Constant5/1 -> Sum1/1

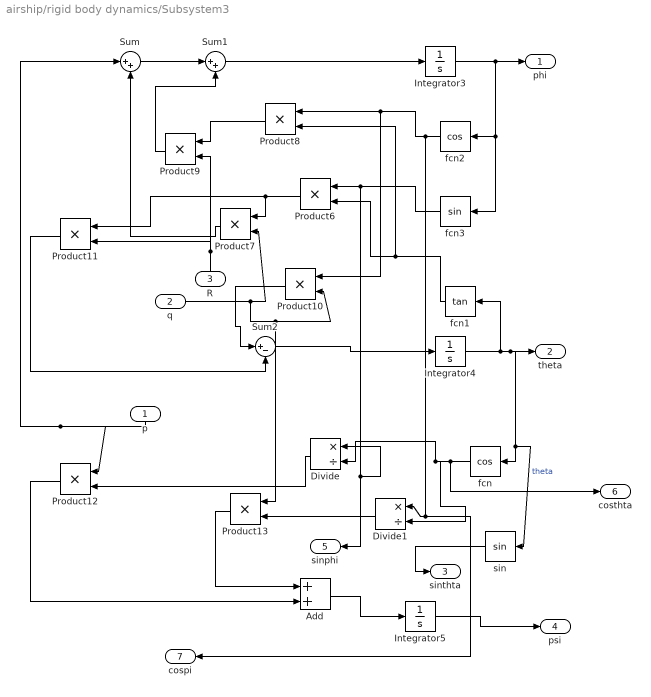
== system airship/rigid body dynamics/Subsystem3 ==
  p : Inport
  q : Inport  Port=2
  R : Inport  Port=3
  Add : Sum  OutDataType=fixdt(1, 16)  OutScaling=2^-10
  Divide : Product  Inputs=*/  OutDataType=fixdt(1, 16)  OutScaling=2^-10
  Divide1 : Product  Inputs=*/  OutDataType=fixdt(1, 16)  OutScaling=2^-10
  Integrator3 : Integrator
  Integrator4 : Integrator
  Integrator5 : Integrator
  Product{6..13} (8 alike) : Product  OutDataType=fixdt(1, 16)  OutScaling=2^0  RndMeth=Zero
  Sum : Sum  Inputs=|++  OutDataType=fixdt(1, 16)  OutScaling=2^0
  Sum1 : Sum  Inputs=|++  OutDataType=fixdt(1, 16)  OutScaling=2^0
  Sum2 : Sum  Inputs=|+-  OutDataType=fixdt(1, 16)  OutScaling=2^0
  fcn : Trigonometry  Operator=cos
  fcn1 : Trigonometry  Operator=tan
  fcn2 : Trigonometry  Operator=cos
  fcn3 : Trigonometry
  sin : Trigonometry
  phi : Outport  OutDataType=fixdt(1, 16)  OutScaling=2^0
  theta : Outport  Port=2  OutDataType=fixdt(1, 16)  OutScaling=2^0
  sinthta : Outport  Port=3  OutDataType=fixdt(1, 16)  OutScaling=2^0
  psi : Outport  Port=4  OutDataType=fixdt(1, 16)  OutScaling=2^0
  sinphi : Outport  Port=5  OutDataType=fixdt(1, 16)  OutScaling=2^0
  costhta : Outport  Port=6  OutDataType=fixdt(1, 16)  OutScaling=2^0
  cospi : Outport  Port=7  OutDataType=fixdt(1, 16)  OutScaling=2^0
  wires:
  Sum/1 -> Sum1/1
  Sum1/1 -> Integrator3/1
  Integrator3/1 -> phi/1, fcn2/1, fcn3/1
  fcn2/1 -> Product8/1, Product10/1, cospi/1, Divide1/1
  fcn3/1 -> Product6/1, sinphi/1, Divide/1
  fcn1/1 -> Product6/2, Product8/2
  Product10/1 -> Sum2/1
  Sum2/1 -> Integrator4/1
  Integrator4/1 -> fcn1/1, theta/1, fcn/1, sin/1  "theta"
  Product8/1 -> Product9/1
  Product9/1 -> Sum1/2
  Product6/1 -> Product11/1, Product7/1
  Product7/1 -> Sum/2
  Product11/1 -> Sum2/2
  fcn/1 -> Divide/2, Divide1/2, costhta/1
  Divide1/1 -> Product13/2
  Product12/1 -> Add/2
  Product13/1 -> Add/1
  q/1 -> Product7/2, Product10/2, Product13/1
  Divide/1 -> Product12/2
  sin/1 -> sinthta/1
  Add/1 -> Integrator5/1
  Integrator5/1 -> psi/1
  R/1 -> Product11/2, Product9/2
  p/1 -> Sum/1, Product12/1
